simulink model "C_test"  (R2023b)
settings: Solver=VariableStepAuto  StartTime=0.0  StopTime=30  RelTol=1e-3
libraries: simulink x4, robotmobilelib x1
settings Model: Creator=rubencruzgonzalez  LastModifiedBy=rubencruzgonzalez
settings DataIOCC: SaveOutput=off  SaveTime=off
settings OptimizationCC: DefaultParameterBehavior=Inlined

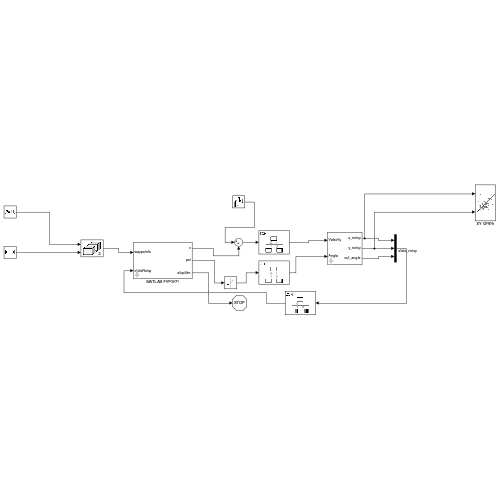
[thumbnail: Simulink's stored preview of the top-level diagram]
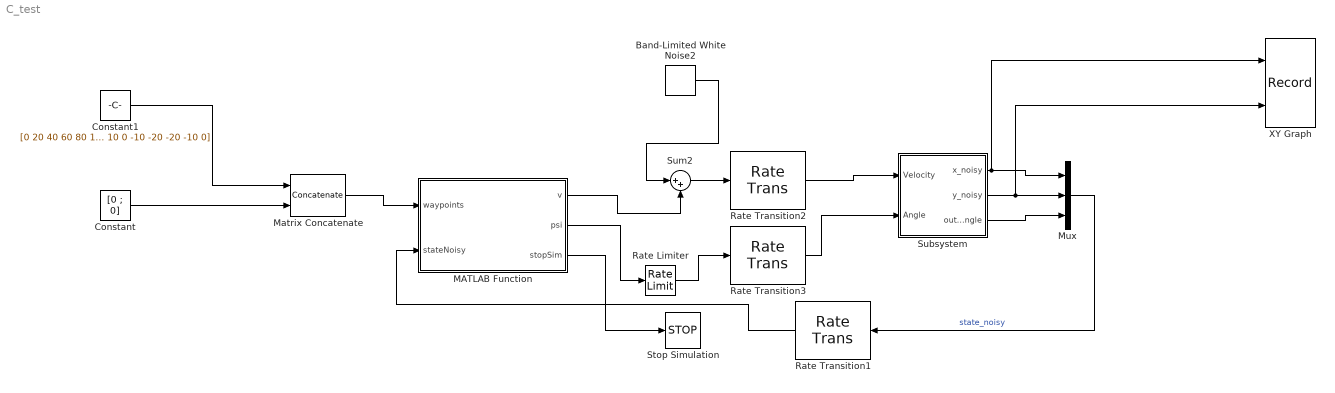
== system C_test ==
  Band-Limited White Noise2 : simulink/Sources/Band-Limited White Noise  Tag=noise_x  Cov=[0.00001]  Ts=1/100000  seed=[23341]
  Constant : Constant  Value=[0 ; 0]
  Constant1 : Constant  Value=[0 20 40 60 80 100 120 140 160 180 200;0 10 20 20 10 0 -10 -20 -20 -10 0]
  MATLAB Function : Subsystem
      mask help: Simulink:masks:GenSFuncDesc_MD
      mask Help: eval('feval(''rtwprivate'',''rtwhelpview'',''rtw_sfcn_block'')');
  Matrix Concatenate : Concatenate  Mode=Multidimensional array  ConcatenateDimension=2
  Mux : Mux  Inputs=3
  Rate Limiter : RateLimiter  RisingSlewLimit=pi/4  FallingSlewLimit=-pi/4  SampleTimeMode=inherited
  Rate Transition1 : RateTransition  OutPortSampleTime=1/100
  Rate Transition2 : RateTransition  OutPortSampleTime=1/1000
  Rate Transition3 : RateTransition  OutPortSampleTime=1/1000
  Stop Simulation : Stop
  Subsystem : Subsystem
  Sum2 : Sum  Inputs=|++
  XY Graph : Record  FileSettingsInternal="{\"entries\":[{\"content\":{\"excelSettings\":{\"content\":{},\"type\":\"Streamout.ExcelSettings\"}},\"type\":\"Streamout.FileSettingStorage\",\"uuid\":\"\"}],\"packageUris\":[\"http:\\/\\/schema.mathworks.com\\/mf0\\/streamout_blocks\\/R2020a\"],\"version\":\"1.0\"}"  Layout=[1 1]  SignalsInternal="{\"entries\":[{\"content\":{\"signals\":[{\"content\":{\"blockPath\":[],\"dimensions\":[1],\"domain\":\"\",\"lineColor\":\"#a2142f\",\"plots\":[1],\"port\":1,\"sid\":[\"\"],\"signalID\":27,\"signalName\":\"Subsystem:1\"},\"type\":\"RecordBlkView.Signal\",\"uuid\":\"\"},{\"content\":{\"blockPath\":[],\"dimensions\":[1],\"domain\":\"\",\"lineColor\":\"#139fff\",\"plots\":[1],\"port\":2,\"sid\":[\"\"],\"signalID\":31,\"signalName\":\"Subsystem:2\"},\"type\":\"RecordBlkView.Signal\",\"uuid\":\"\"}]},\"type\":\"RecordBlkView.InputSignals\",\"uuid\":\"\"}],\"packageUris\":[\"http:\\/\\/schema.mathworks.com\\/mf0\\/streamout_blocks\\/R2020a\"],\"version\":\"1.0\"}"  VisualizationBindings="{\"xyplotplugin\":{\"info\":[{\"series\":[{\"bindingParametersList\":[{\"parameter\":\"X-Axis\",\"signalID\":27,\"signalName\":\"Subsystem:1\"},{\"parameter\":\"Y-Axis\",\"signalID\":31,\"signalName\":\"Subsystem:2\"}],\"seriesID\":486}],\"subplotID\":1}]}}"  CompatibilityTag=XY
  wires:
  Sum2/1 -> Rate Transition2/1
  Subsystem/2(y_noisy) -> XY Graph/2, Mux/2
  Rate Transition2/1 -> Subsystem/1(Velocity)
  MATLAB Function/2(psi) -> Rate Limiter/1
  MATLAB Function/1(v) -> Sum2/2
  Mux/1 -> Rate Transition1/1  "state_noisy"
  Rate Transition3/1 -> Subsystem/2(Angle)
  MATLAB Function/3(stopSim) -> Stop Simulation/1
  Band-Limited White Noise2/1 -> Sum2/1
  Subsystem/3(out_angle) -> Mux/3
  Rate Transition1/1 -> MATLAB Function/2(stateNoisy)
  Rate Limiter/1 -> Rate Transition3/1
  Subsystem/1(x_noisy) -> XY Graph/1, Mux/1
  Matrix Concatenate/1 -> MATLAB Function/1(waypoints)
  Constant1/1 -> Matrix Concatenate/1
  Constant/1 -> Matrix Concatenate/2

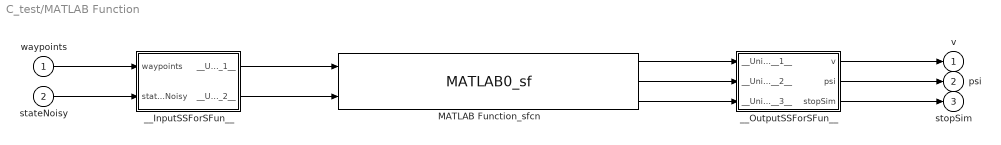
== system C_test/MATLAB Function ==
  waypoints : Inport
  stateNoisy : Inport  Port=2
  MATLAB Function_sfcn : S-Function  FunctionName=MATLAB0_sf  SFunctionModules=""  SFunctionDeploymentMode=off  EnableBusSupport=off  mask{rtw_sf_name=MATLAB0_sf, showVar=off}
      mask prompts: rtw_sf_name "Simulink:masks:GenSFuncName_MP"; showVar "Simulink:masks:GenSFuncShowModuleList_MP"
      mask help: Simulink:masks:GenSFuncDesc_MD
      mask init:
      | displist = '';
      | if ~strcmp(get_param(gcb, 'FunctionName'), rtw_sf_name);
      |   set_param(gcb, 'FunctionName', rtw_sf_name);
      | end
      | % Check if we are generating code
      | rtw_mode = false;
      | if strcmpi(get_param(bdroot(gcb),'SimulationStatus'),'Initializing')
      | 	rtw_mode = strcmpi(get_param(bdroot(gcb),'BuildingRTWCode'),'on') && ...
      | 		~strcmpi(get_param(bdroot(gcb),'TargetStyle'),'SimulationTarget');
      | end
      | if showVar || rtw_mode
      | 	if exist('rtwsfunc') == 2 | exist('rtwsfunc') == 6
      | 		tmplist = rtwsfunc(rtw_sf_name,gcb);
      | 		tmplist = DAStudio.message('Simulink:masks:GenSFuncListOfModules_IC', tmplist);
      | 	elseif showVar
      | 		tmplist1 = DAStudio.message('Simulink:masks:GenSFuncListOfModules_IC', '');
      |         tmplist2 = DAStudio.message('Simulink:masks:GenSFuncNotLicensed_IC');
      |         tmplist = [tmplist1 tmplist2];
      |  	end
      | end
      | if showVar
      |   displist = tmplist;
      | end
      settings: CopyFcn=|
      | if ~strcmp(get_param(gcb,'Linkstatus'),'none') && ...
      | ~strcmp(get_param(gcb,'Linkstatus'),'implicit')
      |   set_param(gcb,'LinkStatus','none');
      | end
      mask Help: eval('feval(''rtwprivate'',''rtwhelpview'',''rtw_sfcn_block'')');
      mask Display:
      | port_label('input',1,'waypoints');
      | port_label('input',2,'stateNoisy');
      | port_label('output',1,'v');
      | port_label('output',2,'psi');
      | port_label('output',3,'stopSim');
  __InputSSForSFun__ : Subsystem
  __OutputSSForSFun__ : Subsystem
  v : Outport
  psi : Outport  Port=2
  stopSim : Outport  Port=3
  wires:
  waypoints/1 -> __InputSSForSFun__/1(waypoints)
  stateNoisy/1 -> __InputSSForSFun__/2(stateNoisy)
  __InputSSForSFun__/1(__UniqueOutportName__1__) -> MATLAB Function_sfcn/1
  __InputSSForSFun__/2(__UniqueOutportName__2__) -> MATLAB Function_sfcn/2
  MATLAB Function_sfcn/1 -> __OutputSSForSFun__/1(__UniqueInportName__1__)
  MATLAB Function_sfcn/2 -> __OutputSSForSFun__/2(__UniqueInportName__2__)
  MATLAB Function_sfcn/3 -> __OutputSSForSFun__/3(__UniqueInportName__3__)
  __OutputSSForSFun__/1(v) -> v/1
  __OutputSSForSFun__/2(psi) -> psi/1
  __OutputSSForSFun__/3(stopSim) -> stopSim/1

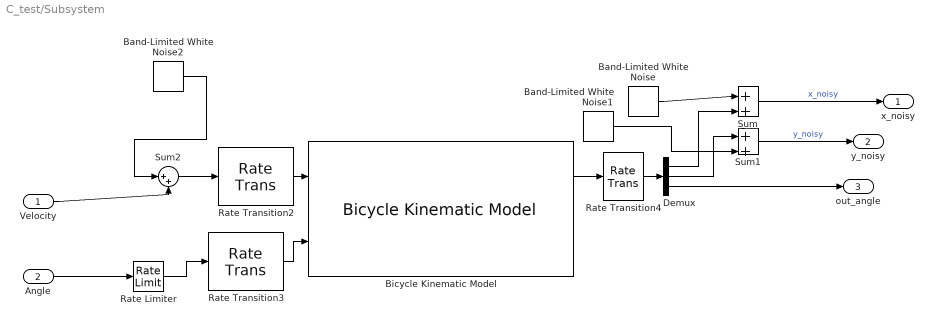
== system C_test/Subsystem ==
  Velocity : Inport
  Angle : Inport  Port=2
  Band-Limited White Noise : simulink/Sources/Band-Limited White Noise  Tag=noise_x  Cov=[0.00001]  Ts=1/100  seed=[23341]
  Band-Limited White Noise1 : simulink/Sources/Band-Limited White Noise  Tag=noise_y  Cov=[0.00001]  Ts=1/100  seed=[23341]
  Band-Limited White Noise2 : simulink/Sources/Band-Limited White Noise  Tag=noise_x  Cov=[0.0001]  Ts=1/100000  seed=[23341]
  Bicycle Kinematic Model : robotmobilelib/Bicycle Kinematic Model  VehicleInputs=Vehicle Speed & Steering Angle  WheelBase=1  VehicleSpeedRange=[0 30]  MaxSteeringAngle=pi/4  InitialState=[0; 0; 0]  SimulateUsing=Code generation
  Demux : Demux  Outputs=3
  Rate Limiter : RateLimiter  RisingSlewLimit=pi/4  FallingSlewLimit=-pi/4  SampleTimeMode=inherited
  Rate Transition2 : RateTransition  OutPortSampleTime=1/1000
  Rate Transition3 : RateTransition  OutPortSampleTime=1/1000
  Rate Transition4 : RateTransition  OutPortSampleTime=1/1000
  Sum : Sum  Inputs=|++
  Sum1 : Sum  Inputs=|++
  Sum2 : Sum  Inputs=|++
  x_noisy : Outport
  y_noisy : Outport  Port=2
  out_angle : Outport  Port=3
  wires:
  Rate Transition2/1 -> Bicycle Kinematic Model/1
  Rate Limiter/1 -> Rate Transition3/1
  Band-Limited White Noise1/1 -> Sum1/2
  Rate Transition3/1 -> Bicycle Kinematic Model/2
  Demux/2 -> Sum1/1
  Band-Limited White Noise/1 -> Sum/1
  Demux/3 -> out_angle/1
  Sum1/1 -> y_noisy/1  "y_noisy"
  Sum2/1 -> Rate Transition2/1
  Band-Limited White Noise2/1 -> Sum2/1
  Sum/1 -> x_noisy/1  "x_noisy"
  Rate Transition4/1 -> Demux/1
  Angle/1 -> Rate Limiter/1
  Demux/1 -> Sum/2
  Bicycle Kinematic Model/1 -> Rate Transition4/1
  Velocity/1 -> Sum2/2

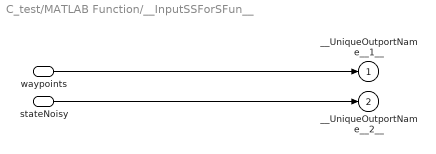
== system C_test/MATLAB Function/__InputSSForSFun__ ==
  waypoints : Inport
  stateNoisy : Inport  Port=2
  __UniqueOutportName__1__ : Outport
  __UniqueOutportName__2__ : Outport  Port=2
  wires:
  waypoints/1 -> __UniqueOutportName__1__/1
  stateNoisy/1 -> __UniqueOutportName__2__/1

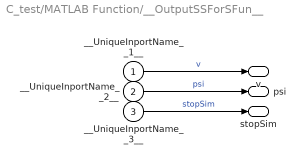
== system C_test/MATLAB Function/__OutputSSForSFun__ ==
  __UniqueInportName__1__ : Inport
  __UniqueInportName__2__ : Inport  Port=2
  __UniqueInportName__3__ : Inport  Port=3
  v : Outport
  psi : Outport  Port=2
  stopSim : Outport  Port=3
  wires:
  __UniqueInportName__1__/1 -> v/1  "v"
  __UniqueInportName__2__/1 -> psi/1  "psi"
  __UniqueInportName__3__/1 -> stopSim/1  "stopSim"
